simulink model "parte5_eje2_GEPs"  (R2017b)
settings: Solver=ode45  StartTime=0.0  StopTime=10  RelTol=1e-3  EnableMultiTasking=on
model workspace (MAT data in the model file):
  D = 0
  F = 60
  H = 6.5
  KAe = 200
  T1e = 1
  T1p = 0.648927607606
  T2e = 10
  T2p = 0.216309202535
  T3 = 1.40659340659
  T3p = 0.648927607606
  T4p = 0.216309202535
  Tee = 0.01
  Tre = 0.01
  Twp = 10
  k1 = 2.21807614913
  k2 = 3.1205207777
  k3 = 0.175824175824
  k4 = 4.68078116655
  k5 = -0.130081858844
  k6 = 0.00523421739465
values from neighbouring files (symbols this model uses):
  K2 = 0.95567    [parte5_ej2_GEPs_data0228.m]    (also in parte5_eje2_sintonizacionPSS.m = Lads/(Lads+Lfd)*(RT/D*eqo+(XTQ*(xq-xpd)/D+1)*iqo))
  K3 = 0.34284    [parte5_ej2_GEPs_data0228.m]    (also in parte5_eje2_sintonizacionPSS.m = (Lads+Lfd)/Ladu*1/(1+XTQ/D*(xd+xpd)))
  K6 = 0.070874    [parte5_ej2_GEPs_data0228.m]    (also in parte5_eje2_sintonizacionPSS.m = xe*(vqo/Et)/(xe+xpd))
  KA = 200    [parte5_eje2_sintonizacionPSS.m]
  TA = 0.1    [parte5_eje2_sintonizacionPSS.m]
  Tr = 0.01    [parte5_ej2_GEPs_data0228.m]    (also in parte5_eje2_sintonizacionPSS.m)
settings Model: Creator=ramos  LastModifiedBy=cjuar
settings DataIOCC: LimitDataPoints=on  SaveFormat=Array  SignalLoggingSaveFormat=ModelDataLogs
settings OptimizationCC: ExpressionDepthLimit=2147483647  LifeSpan=inf
settings DebuggingCC: UnderspecifiedInitializationDetection=Classic  MergeDetectMultiDrivingBlocksExec=none  SolverPrmCheckMsg=warning  FcnCallInpInsideContextMsg=warning  StateNameClashWarn=warning  SFUnexpectedBacktrackingDiag=warning  SFNoUnconditionalDefaultTransitionDiag=warning  SFExecutionAtInitializationDiag=none
settings HardwareCC: ProdBitPerPointer=32  ProdBitPerSizeT=32  ProdBitPerPtrDiffT=32  ProdLargestAtomicFloat=None  ProdIntDivRoundTo=Undefined  ProdEndianess=Unspecified  ProdWordSize=32  ProdHWDeviceType=32-bit Generic
settings ModelReferenceCC: PropagateSignalLabelsOutOfModel=off
settings CodeAppCC: StateflowObjectComments=on
settings GRTTargetCC: TargetLangStandard=C89/C90 (ANSI)  GeneratePreprocessorConditionals=Disable all  CombineOutputUpdateFcns=off  GRTInterface=on
settings ConfigComp: CovMetricSettings=dw  CovHtmlReporting=on  CovSaveCumulativeToWorkspaceVar=on  CovSaveSingleToWorkspaceVar=on  CovExternalEMLEnable=off

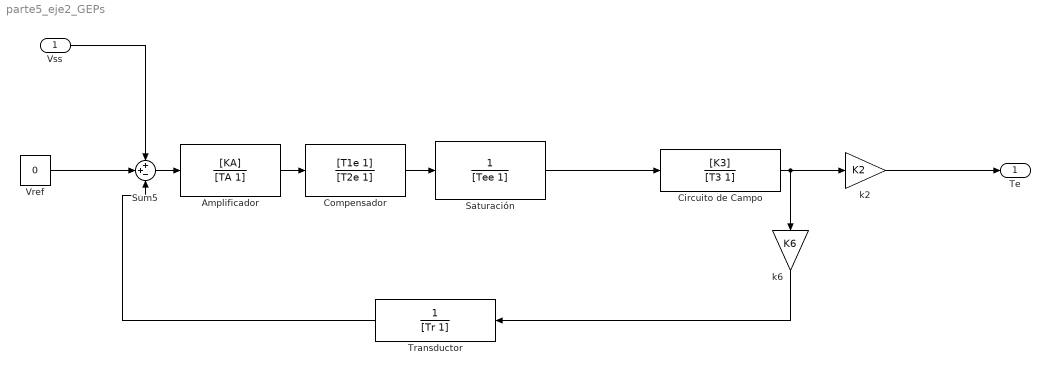
== system parte5_eje2_GEPs ==
  Vss : Inport
  Amplificador : TransferFcn  Numerator=[KA]  Denominator=[TA 1]
  Circuito de Campo : TransferFcn  Numerator=[K3]  Denominator=[T3 1]
  Compensador : TransferFcn  Numerator=[T1e 1]  Denominator=[T2e 1]
  Saturación : TransferFcn  Denominator=[Tee 1]
  Sum5 : Sum  Inputs=++-
  Transductor : TransferFcn  Denominator=[Tr 1]
  Vref : Constant  Value=0
  k2 : Gain  Gain=K2
  k6 : Gain  Gain=K6
  Te : Outport
  wires:
  Circuito de Campo/1 -> k2/1, k6/1
  Saturación/1 -> Circuito de Campo/1
  k6/1 -> Transductor/1
  Vss/1 -> Sum5/1
  Transductor/1 -> Sum5/3
  Compensador/1 -> Saturación/1
  Sum5/1 -> Amplificador/1
  Amplificador/1 -> Compensador/1
  k2/1 -> Te/1
  Vref/1 -> Sum5/2
